simulink model "STP_CTL"  (R2019a)
settings: Solver=FixedStepDiscrete  StartTime=0.0  StopTime=inf  FixedStep=0.001  RelTol=1e-3  EnableMultiTasking=on
undefined symbols (not defined in the file): HIL
libraries: quarc_library x6
settings Model: SimulationMode=external  ExtModeTrigDuration=10000  Creator=21nww3  LastModifiedBy=21nww3
settings SolverCC: PositivePriorityOrder=on
settings RTWCC: SystemTargetFile=quarc_win64.tlc  TemplateMakefile=quarc_default_tmf  Description=QUARC Win64 Target
settings STFCustomTargetCC: TargetPreCompLibLocation=C:\PROGRA~3\QUARC\lib\2019a\win64\release  TargetLangStandard=C99 (ISO)  ConcurrentExecutionCompliant=on  SystemTargetFile=quarc_win64.tlc
settings GRTTargetCC: TargetPreCompLibLocation=C:\PROGRA~3\QUARC\lib\2019a\win64\release  ParMdlRefBuildCompliant=off  CompOptLevelCompliant=off  CombineOutputUpdateFcns=off  MatFileLogging=off  CPPClassGenCompliant=off  GRTInterface=on  UseToolchainInfoCompliant=off  ExtMode=on  ExtModeMexFile=quarc_comm

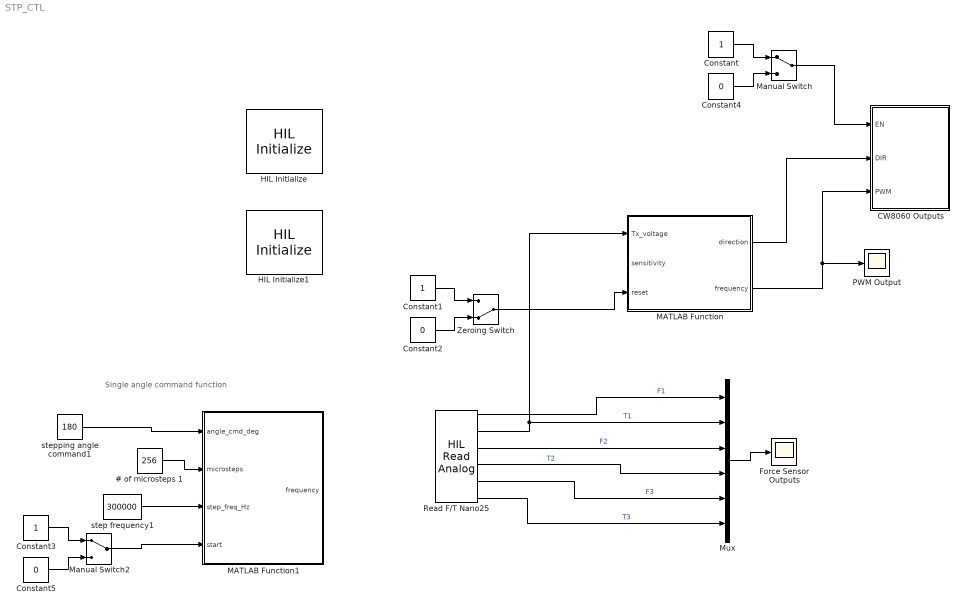
== system STP_CTL ==
  note: Single angle command function
  # of microsteps 1 : Constant  Value=256
  CW8060 Outputs : Subsystem
  Constant : Constant
  Constant1 : Constant
  Constant2 : Constant  Value=0
  Constant3 : Constant
  Constant4 : Constant  Value=0
  Constant5 : Constant  Value=0
  Force Sensor Outputs : Scope
  HIL Initialize : quarc_library/Data Acquisition/Generic/Configuration/HIL Initialize  object_name=HIL-1  board_type=q8  board_number=0  board_options=""  exclusive=off  active=on  hardware_clocks=[0:1]  clock_modes=[1 0]  initial_clock_frequencies=[]  set_clock_params_at_start=on  set_clock_params_at_switch_in=off  set_clock_frequencies_at_start=off  set_clock_frequencies_at_switch_in=off  analog_input_channels=[0:7]  analog_input_configurations=[]  analog_input_maximums=10  analog_input_minimums=-10  set_analog_input_params_at_start=off  set_analog_input_params_at_switch_in=off  analog_output_channels=[0:7]  analog_output_maximums=[10]  analog_output_minimums=[-10]  initial_analog_outputs=[0]  final_analog_outputs=[0]  watchdog_analog_outputs=0  set_analog_output_params_at_start=on  set_analog_output_params_at_switch_in=off  set_analog_outputs_at_start=on  set_analog_outputs_at_switch_in=off  set_analog_outputs_at_terminate=on  set_analog_outputs_at_switch_out=off  set_analog_outputs_on_watchdog=off  digital_input_channels=[]  digital_output_channels=[1:2]  digital_output_configuration=[]  initial_digital_outputs=[0]  final_digital_outputs=[0]  watchdog_digital_outputs=[2]  set_digital_output_params_at_start=off  set_digital_output_params_at_switch_in=off  set_digital_outputs_at_start=on  set_digital_outputs_at_switch_in=off  set_digital_outputs_at_terminate=on  set_digital_outputs_at_switch_out=off  set_digital_outputs_on_watchdog=off  encoder_channels=[0:7]  quadrature=[4]  encoder_filter_frequency=(1/120e-9)/1  initial_encoder_counts=[0]  set_encoder_params_at_start=on  set_encoder_params_at_switch_in=off  set_encoder_counts_at_start=on  set_encoder_counts_at_switch_in=off  pwm_channels=[0]  pwm_modes=[1]  pwm_frequency=0.5  pwm_configuration=[]  pwm_alignment=[]  pwm_polarity=[]  pwm_leading_deadband=[]  pwm_trailing_deadband=[]  initial_pwm_outputs=[0]  final_pwm_outputs=[0]  watchdog_pwm_outputs=[]  set_pwm_params_at_start=on  set_pwm_params_at_switch_in=off  set_pwm_outputs_at_start=on  set_pwm_outputs_at_switch_in=off  set_pwm_outputs_at_terminate=on  set_pwm_outputs_at_switch_out=off  set_pwm_outputs_on_watchdog=off  other_output_channels=[]  initial_other_outputs=[]  final_other_outputs=[]  watchdog_other_outputs=[]  set_other_outputs_at_start=off  set_other_outputs_at_switch_in=off  set_other_outputs_at_terminate=off  set_other_outputs_at_switch_out=off  set_other_outputs_on_watchdog=off
  HIL Initialize1 : quarc_library/Data Acquisition/Generic/Configuration/HIL Initialize  object_name=HIL-2  board_type=ni_pci_6034e  board_number=0  board_options=terminal_board=e_series  exclusive=off  active=on  hardware_clocks=[]  clock_modes=[]  initial_clock_frequencies=[]  set_clock_params_at_start=off  set_clock_params_at_switch_in=off  set_clock_frequencies_at_start=off  set_clock_frequencies_at_switch_in=off  analog_input_channels=[0:15]  analog_input_configurations=[]  analog_input_maximums=10  analog_input_minimums=-10  set_analog_input_params_at_start=on  set_analog_input_params_at_switch_in=off  analog_output_channels=[]  analog_output_maximums=[]  analog_output_minimums=[]  initial_analog_outputs=[]  final_analog_outputs=[]  watchdog_analog_outputs=[]  set_analog_output_params_at_start=off  set_analog_output_params_at_switch_in=off  set_analog_outputs_at_start=off  set_analog_outputs_at_switch_in=off  set_analog_outputs_at_terminate=off  set_analog_outputs_at_switch_out=off  set_analog_outputs_on_watchdog=off  digital_input_channels=[]  digital_output_channels=[]  digital_output_configuration=[]  initial_digital_outputs=[1]  final_digital_outputs=[1]  watchdog_digital_outputs=[]  set_digital_output_params_at_start=off  set_digital_output_params_at_switch_in=off  set_digital_outputs_at_start=on  set_digital_outputs_at_switch_in=off  set_digital_outputs_at_terminate=on  set_digital_outputs_at_switch_out=off  set_digital_outputs_on_watchdog=off  encoder_channels=[]  quadrature=[0]  encoder_filter_frequency=[]  initial_encoder_counts=[0]  set_encoder_params_at_start=off  set_encoder_params_at_switch_in=off  set_encoder_counts_at_start=on  set_encoder_counts_at_switch_in=off  pwm_channels=[]  pwm_modes=[0]  pwm_frequency=20e6/4096  pwm_configuration=[]  pwm_alignment=[]  pwm_polarity=[]  pwm_leading_deadband=[]  pwm_trailing_deadband=[]  initial_pwm_outputs=[0]  final_pwm_outputs=[0]  watchdog_pwm_outputs=[]  set_pwm_params_at_start=on  set_pwm_params_at_switch_in=off  set_pwm_outputs_at_start=on  set_pwm_outputs_at_switch_in=off  set_pwm_outputs_at_terminate=on  set_pwm_outputs_at_switch_out=off  set_pwm_outputs_on_watchdog=off  other_output_channels=[]  initial_other_outputs=[]  final_other_outputs=[]  watchdog_other_outputs=[]  set_other_outputs_at_start=off  set_other_outputs_at_switch_in=off  set_other_outputs_at_terminate=off  set_other_outputs_at_switch_out=off  set_other_outputs_on_watchdog=off
  MATLAB Function : MATLAB Function  TreatAsAtomicUnit=on
  MATLAB Function1 : MATLAB Function  TreatAsAtomicUnit=on
  Manual Switch : ManualSwitch
  Manual Switch2 : ManualSwitch
  Mux : Mux  Inputs=6
  PWM Output : Scope
      settings: Tag=PWM Output
  Read F/T Nano25 : quarc_library/Data Acquisition/Generic/Immediate I//O/HIL Read Analog  object_name=HIL-2  channels=[0:5]  sample_time=qc_get_step_size  active=on  vector_output=off
  Zeroing Switch : ManualSwitch  CurrentSetting=0
  step frequency1 : Constant  Value=300000
  stepping angle command1 : Constant  Value=180
  wires:
  Manual Switch/1 -> CW8060 Outputs/1(EN)
  MATLAB Function/1(direction) -> CW8060 Outputs/2(DIR)
  MATLAB Function/2(frequency) -> CW8060 Outputs/3(PWM), PWM Output/1
  Constant/1 -> Manual Switch/1
  Constant4/1 -> Manual Switch/2
  Read F/T Nano25/1 -> Mux/1  "F1"
  Read F/T Nano25/2 -> Mux/2, MATLAB Function/1(Tx_voltage)  "T1"
  Read F/T Nano25/3 -> Mux/3  "F2"
  Read F/T Nano25/4 -> Mux/4  "T2"
  Read F/T Nano25/5 -> Mux/5  "F3"
  Read F/T Nano25/6 -> Mux/6  "T3"
  Mux/1 -> Force Sensor Outputs/1
  Manual Switch2/1 -> MATLAB Function1/4(start)
  stepping angle command1/1 -> MATLAB Function1/1(angle_cmd_deg)
  Constant3/1 -> Manual Switch2/1
  # of microsteps 1/1 -> MATLAB Function1/2(microsteps)
  step frequency1/1 -> MATLAB Function1/3(step_freq_Hz)
  Constant5/1 -> Manual Switch2/2
  Constant2/1 -> Zeroing Switch/2
  Constant1/1 -> Zeroing Switch/1
  Zeroing Switch/1 -> MATLAB Function/3(reset)

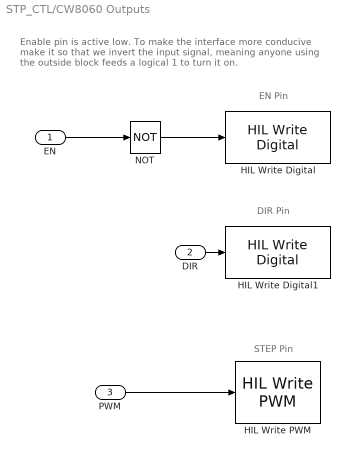
== system STP_CTL/CW8060 Outputs ==
  note: Enable pin is active low. To make the interface more conducive
      | make it so that we invert the input signal, meaning anyone
      | using the outside block feeds a logical 1 to turn it on.
  note: EN Pin
  note: DIR Pin
  note: STEP Pin
  EN : Inport
  DIR : Inport  Port=2
  PWM : Inport  Port=3
  HIL Write Digital : quarc_library/Data Acquisition/Generic/Immediate I//O/HIL Write Digital  object_name=HIL-1  channels=1  sample_time=-1  active=off  vector_input=off
      settings: SourceProductName=QUARC Targets
  HIL Write Digital1 : quarc_library/Data Acquisition/Generic/Immediate I//O/HIL Write Digital  object_name=HIL-1  channels=2  sample_time=-1  active=off  vector_input=off
      settings: SourceProductName=QUARC Targets
  HIL Write PWM : quarc_library/Data Acquisition/Generic/Immediate I//O/HIL Write PWM  object_name=HIL-1  channels=[0]  sample_time=-1  active=off  vector_input=off
      settings: AttributesFormatString=(%<object_name>)  SourceProductName=QUARC Targets
  NOT : Logic  Operator=NOT  IconShape=distinctive  AllPortsSameDT=off  OutDataTypeStr=boolean
  wires:
  DIR/1 -> HIL Write Digital1/1
  PWM/1 -> HIL Write PWM/1
  EN/1 -> NOT/1
  NOT/1 -> HIL Write Digital/1

== matlab function STP_CTL/MATLAB Function1 ==
  data: angle_cmd_deg input; microsteps input; step_freq_Hz input; frequency output; start input
function frequency = stepper_angle_cmd(angle_cmd_deg, microsteps, step_freq_Hz, start)
% angle_cmd_deg : desired rotation (deg)
% microsteps    : microstepping multiplier (1, 2, 4, 8, 16, etc.)
% step_freq_Hz  : step frequency in Hz
% start         : boolean (1 = start move)
% frequency     : output frequency in Hz (0 when stopped)

persistent pulses_target time_target time_elapsed active prev_start

% ---- Parameters ----
steps_per_rev = 200;      % full steps per revolution
Ts = 0.001;               % sample time (1 kHz)

% ---- Initialize persistent variables ----
if isempty(active)
    pulses_target = 0;
    time_target = 0;
    time_elapsed = 0;
    active = 0;
    prev_start = 0;
end

% ---- Detect rising edge on start signal ----
start_edge = (start && ~prev_start);
prev_start = start;

% ---- Start new move on rising edge ----
if start_edge
    % Calculate total microsteps needed
    total_steps = steps_per_rev * microsteps;
    pulses_target = abs(round(angle_cmd_deg * total_steps / 360));
    time_target = pulses_target / step_freq_Hz;
    time_elapsed = 0;
    active = 1;
end

% ---- Motion logic ----
if active
    time_elapsed = time_elapsed + Ts;
    if time_elapsed >= time_target
        frequency = 0;
        active = 0;
    else
        frequency = step_freq_Hz;
    end
else
    frequency = 0;
end
end

== matlab function STP_CTL/MATLAB Function ==
  data: direction output; Tx_voltage input; sensitivity input; frequency output; reset input
function [direction, frequency] = force_control_stepper(Tx_voltage, sensitivity, reset)
% Tx_voltage  : Raw voltage reading from torque sensor channel
% microsteps  : Microstepping multiplier (1, 2, 4, 8, 16, etc.)
% reset       : Set to 1 to re-zero the sensor
% frequency   : Output frequency 0-30000 Hz
% direction   : Direction signal (0 or 1)

persistent Tx_zero is_zeroed

% ---- Parameters ----
max_freq = 30000;    % Maximum frequency in Hz at microsteps=1
voltage_range = 1.0;      % 0-1V range for full scale

% ---- Initialize persistent variables ----
if isempty(is_zeroed)
    Tx_zero = 0;
    is_zeroed = false;
end

% ---- Manual reset / re-zero ----
if reset
    Tx_zero = Tx_voltage;
    is_zeroed = true;
    frequency = 0;
    direction = 1;
    return;
end

% ---- Auto-zero on first reading ----
if ~is_zeroed
    Tx_zero = Tx_voltage;
    is_zeroed = true;
end

% ---- Calculate zeroed voltage ----
Tx_zeroed = Tx_voltage - Tx_zero;

% ---- Determine direction ----
if Tx_zeroed >= 0
    direction = 1;  % Positive direction
else
    direction = 0;  % Negative direction
end

% ---- Calculate frequency (absolute value, 0-1V → 0-30000Hz) ----
Tx_abs = abs(Tx_zeroed) * sensitivity;

% Clamp to voltage range
if Tx_abs > voltage_range
    Tx_abs = voltage_range;
end

% Map voltage to frequency linearly
frequency = (Tx_abs / voltage_range) * max_freq;

end
